simulink model "MATLABProperty_harness"  (R2021b)
settings: Solver=FixedStepDiscrete  StartTime=0  StopTime=0.01  FixedStep=0.01  RelTol=1e-3  EnableMultiTasking=on
PreLoadFcn:
  | load sldvdemo_sbrBusDef
undefined symbols (not defined in the file or in its folder): sigbuilder_block
libraries: simulink x1
settings Model: SldvGeneratedHarnessModel=TestUnitModel=MATLABProperty|  DVExtractedSubsystem=MATLAB Property  Creator=Alessandro  LastModifiedBy=Alessandro
settings SolverCC: AlgebraicLoopSolver=TrustRegion
settings DataIOCC: LimitDataPoints=on  SaveFormat=StructureWithTime  ReturnWorkspaceOutputs=off
settings OptimizationCC: BlockReduction=off  ExpressionFolding=off  ExpressionDepthLimit=2147483647  InitFltsAndDblsToZero=on  LifeSpan=1  EfficientTunableParamExpr=on
settings DebuggingCC: UnderspecifiedInitializationDetection=Classic  MergeDetectMultiDrivingBlocksExec=none  SolverPrmCheckMsg=warning  InheritedTsInSrcMsg=none  FcnCallInpInsideContextMsg=warning  FrameProcessingCompatibilityMsg=none  AllowSymbolicDim=off  StateNameClashWarn=warning  SymbolicDimsDataTypeCodeGenerationDiagnostic=none  SFUnexpectedBacktrackingDiag=warning  SFNoUnconditionalDefaultTransitionDiag=warning  SFExecutionAtInitializationDiag=none  SFMachineParentedDataDiag=warning  ArithmeticOperatorsInVariantConditions=warning
settings HardwareCC: ProdBitPerPointer=32  ProdBitPerSizeT=32  ProdBitPerPtrDiffT=32  ProdLargestAtomicFloat=None  ProdIntDivRoundTo=Undefined  ProdEndianess=Unspecified  ProdWordSize=32  ProdHWDeviceType=32-bit Generic
settings ModelReferenceCC: PropagateSignalLabelsOutOfModel=off
settings SFSimCC: SimUseLocalCustomCode=off  SimParseCustomCode=off  MATLABDynamicMemAlloc=off  CustomCodeUndefinedFunction=UseInterfaceOnly
settings RTWCC: Description=Real-Time Workshop Embedded Coder (no auto configuration)  SystemTargetFile=ert.tlc  TLCOptions=-aAlwaysIncludeCustomSrc=1  GenCodeOnly=on  TemplateMakefile=ert_default_tmf  RTWUseLocalCustomCode=off
settings CodeAppCC: IgnoreCustomStorageClasses=off  CustomSymbolStrType=$N$R$M  CustomSymbolStrModelFcn=$N  StateflowObjectComments=on  InternalIdentifier=Classic
settings ERTTargetCC: MultiwordLength=2048  GenerateSampleERTMain=on  ERTCustomFileTemplate=example_file_process.tlc  ConvertIfToSwitch=off  SuppressUnreachableDefaultCases=off
settings ConfigComp: DVMode=PropertyProving  DVMaxProcessTime=600  DVParameters=on  DVModelCoverageObjectives=MCDC  DVMaxTestCaseSteps=500  DVTestSuiteOptimization=Auto  DVDetectActiveLogic=on  DVSaveHarnessModel=on  DVRebuildModelRepresentation=Always

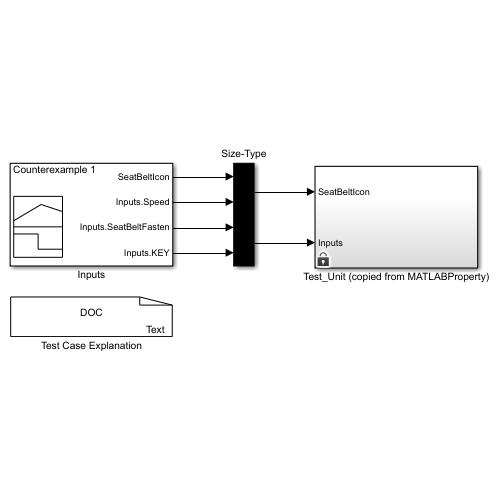
[thumbnail: Simulink's stored preview of the top-level diagram]
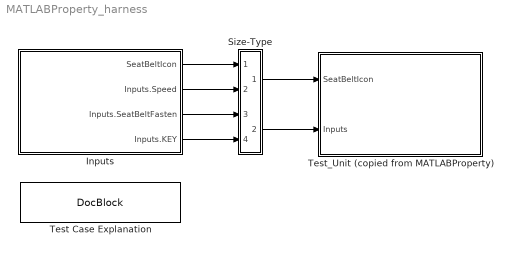
== system MATLABProperty_harness ==
  Inputs : Subsystem  Tag=STV Subsys  LoadFcn=sigbuilder_block('load',[50 50 520 400 ]);  StartFcn=sigbuilder_block('start');  StopFcn=sigbuilder_block('stop');  ClipboardFcn=sigbuilder_block('clipboard');  mask(Sigbuilder block){tuvar=[0:10]}
      mask init:
      | if ~strcmp(get_param(bdroot(gcb),'SimulationStatus'),'stopped'),tuvar = sigbuilder_block('maskInit'); end
      settings: CopyFcn=sigbuilder_block('copy');  DeleteFcn=sigbuilder_block('delete');  ModelCloseFcn=sigbuilder_block('modelClose');  PreSaveFcn=sigbuilder_block('preSave');  PauseFcn=sigbuilder_block('pause');  ContinueFcn=sigbuilder_block('continue');  NameChangeFcn=sigbuilder_block('namechange');  OpenFcn=sigbuilder_block('open');  CloseFcn=sigbuilder_block('close');
      mask Display: plot(0, 0, 100, 100,[2, 2, 32, 32, 2], [68, 8, 8, 68, 68],[32, 2], [38, 38], [32, 19, 2],[53, 60, 44], [32, 17, 17, 2],[16, 16, 31, 31]);txt = getActiveGroup(gcbh);text(2, 100, txt,'verticalAlignment', 'top');
  Size-Type : Subsystem
  Test Case Explanation : simulink/Model-Wide Utilities/DocBlock  DocumentType=Text
  Test_Unit (copied from MATLABProperty) : Subsystem
  wires:
  Inputs/1(SeatBeltIcon) -> Size-Type/1(In1)
  Size-Type/1(Out1) -> Test_Unit (copied from MATLABProperty)/1(SeatBeltIcon)
  Inputs/2(Inputs.Speed) -> Size-Type/2(In2)
  Inputs/3(Inputs.SeatBeltFasten) -> Size-Type/3(In3)
  Inputs/4(Inputs.KEY) -> Size-Type/4(In4)
  Size-Type/2(Out2) -> Test_Unit (copied from MATLABProperty)/2(Inputs)

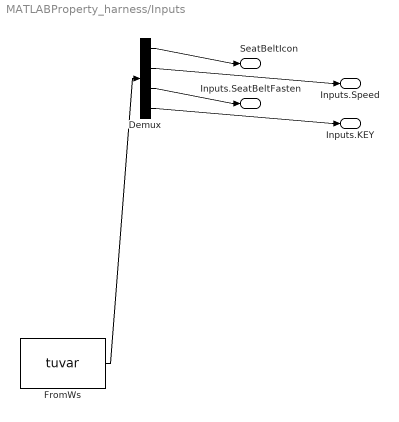
== system MATLABProperty_harness/Inputs ==
  Demux : Demux  Tag=STV Demux
  FromWs : FromWorkspace  Tag=STV FromWs  VariableName=tuvar
      SigBuilderData=|
      | dataSet.timeRange = [0 0.01]
      | dataSet.name = 'Counterexample 1'
      | sbobj.Name = 'Signal Builder'
      | sbobj.Groups.Name = 'Counterexample 1'
      | sbobj.Groups.Signals(1).Name = 'SeatBeltIcon'
      | sbobj.Groups.Signals(1).XData = [0 0.01]
      | sbobj.Groups.Signals(1).YData = [0 0]
      | sbobj.Groups.Signals(2).Name = 'Inputs.Speed'
      | sbobj.Groups.Signals(2).XData = [0 0.01]
      | sbobj.Groups.Signals(2).YData = [13 13]
      | sbobj.Groups.Signals(3).Name = 'Inputs.SeatBeltFasten'
      | sbobj.Groups.Signals(3).XData = [0 0.01]
      | sbobj.Groups.Signals(3).YData = [0 0]
      | sbobj.Groups.Signals(4).Name = 'Inputs.KEY'
      | sbobj.Groups.Signals(4).XData = [0 0.01]
      | sbobj.Groups.Signals(4).YData = [115 115]
      | sbobj.Groups.TimeRange = [0 0.01]
  SeatBeltIcon : Outport  Tag=STV Outport
  Inputs.Speed : Outport  Tag=STV Outport  Port=2
  Inputs.SeatBeltFasten : Outport  Tag=STV Outport  Port=3
  Inputs.KEY : Outport  Tag=STV Outport  Port=4
  wires:
  FromWs/1 -> Demux/1
  Demux/1 -> SeatBeltIcon/1
  Demux/2 -> Inputs.Speed/1
  Demux/3 -> Inputs.SeatBeltFasten/1
  Demux/4 -> Inputs.KEY/1

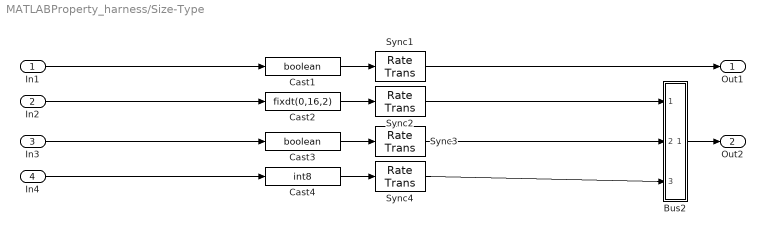
== system MATLABProperty_harness/Size-Type ==
  In1 : Inport
  In2 : Inport  Port=2
  In3 : Inport  Port=3
  In4 : Inport  Port=4
  Bus2 : Subsystem
  Cast1 : DataTypeConversion  OutDataTypeStr=boolean  RndMeth=Nearest  SaturateOnIntegerOverflow=on
  Cast2 : DataTypeConversion  OutDataTypeStr=fixdt(0,16,2)  RndMeth=Nearest  SaturateOnIntegerOverflow=on
  Cast3 : DataTypeConversion  OutDataTypeStr=boolean  RndMeth=Nearest  SaturateOnIntegerOverflow=on
  Cast4 : DataTypeConversion  OutDataTypeStr=int8  RndMeth=Nearest  SaturateOnIntegerOverflow=on
  Sync{1..4} (4 alike) : RateTransition  OutPortSampleTime=[0.01,0]
  Out1 : Outport
  Out2 : Outport  Port=2
  wires:
  In1/1 -> Cast1/1
  Cast1/1 -> Sync1/1
  Sync1/1 -> Out1/1
  In2/1 -> Cast2/1
  Cast2/1 -> Sync2/1
  In3/1 -> Cast3/1
  Cast3/1 -> Sync3/1
  In4/1 -> Cast4/1
  Cast4/1 -> Sync4/1
  Sync2/1 -> Bus2/1(Inputs(1).Speed)
  Sync3/1 -> Bus2/2(Inputs(1).SeatBeltFasten)
  Sync4/1 -> Bus2/3(Inputs(1).KEY)
  Bus2/1(Out) -> Out2/1

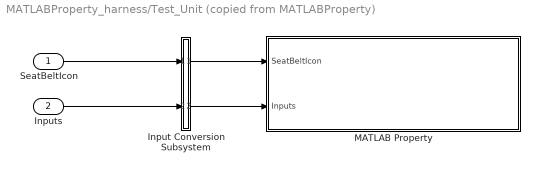
== system MATLABProperty_harness/Test_Unit (copied from MATLABProperty) ==
  SeatBeltIcon : Inport  OutDataTypeStr=boolean  PortDimensions=[1]  SampleTime=0.01  Interpolate=off
  Inputs : Inport  Port=2  OutDataTypeStr=Bus: sbrInputs  PortDimensions=[1]  SampleTime=0.01  Interpolate=off  BusOutputAsStruct=on
  Input Conversion Subsystem : Subsystem  Tag=__SLT_ICS__  Description=|
      | Signal spec.
      | and routing
      settings: AttributesFormatString=%<Description>
  MATLAB Property : MATLAB Function  TreatAsAtomicUnit=on
  wires:
  SeatBeltIcon/1 -> Input Conversion Subsystem/1(Inport_1)
  Inputs/1 -> Input Conversion Subsystem/2(Inport_2)
  Input Conversion Subsystem/1(Outport_1) -> MATLAB Property/1(SeatBeltIcon)
  Input Conversion Subsystem/2(Outport_2) -> MATLAB Property/2(Inputs)

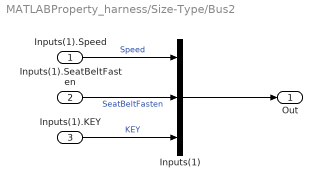
== system MATLABProperty_harness/Size-Type/Bus2 ==
  Inputs(1).Speed : Inport
  Inputs(1).SeatBeltFasten : Inport  Port=2
  Inputs(1).KEY : Inport  Port=3
  Inputs(1) : BusCreator  Inputs=3  OutDataTypeStr=Bus: sbrInputs  NonVirtualBus=on
  Out : Outport
  wires:
  Inputs(1).Speed/1 -> Inputs(1)/1  "Speed"
  Inputs(1).SeatBeltFasten/1 -> Inputs(1)/2  "SeatBeltFasten"
  Inputs(1).KEY/1 -> Inputs(1)/3  "KEY"
  Inputs(1)/1 -> Out/1

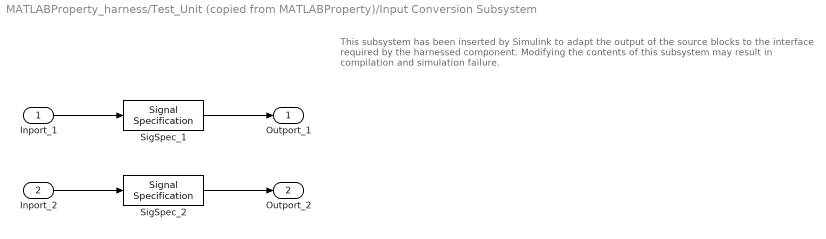
== system MATLABProperty_harness/Test_Unit (copied from MATLABProperty)/Input Conversion Subsystem ==
  note: This subsystem has been inserted by Simulink to adapt the output of the source blocks to the interface required by the harnessed component.
      |  Modifying the contents of this subsystem may result in compilation and simulation failure.
  Inport_1 : Inport
  Inport_2 : Inport  Port=2
  SigSpec_1 : SignalSpecification  OutDataTypeStr=boolean  Dimensions=[1]  SampleTime=0.01
  SigSpec_2 : SignalSpecification  OutDataTypeStr=Bus: sbrInputs  Dimensions=[1]  SampleTime=0.01  BusOutputAsStruct=on
  Outport_1 : Outport
  Outport_2 : Outport  Port=2
  wires:
  Inport_2/1 -> SigSpec_2/1
  SigSpec_2/1 -> Outport_2/1
  Inport_1/1 -> SigSpec_1/1
  SigSpec_1/1 -> Outport_1/1

== matlab function MATLABProperty_harness/Test_Unit (copied from MATLABProperty)/MATLAB Property ==
  data: SeatBeltIcon input boolean; Inputs input sbrInputs
function check_reminder(SeatBeltIcon,Inputs) %#codegen
    % The seat belt light should be active whenever the key is turned on
    % and speed is less than 15 and the seatbelt is not fastened
    activeCond = ((Inputs.KEY ~= 0) && (Inputs.SeatBeltFasten == 0) && ...
                  (Inputs.Speed < 15));
              
    sldv.prove(implies(activeCond,SeatBeltIcon));

function out = implies(cond, result)
    if (cond)
        out = result;
    else
        out = true;
    end
